simulink model "sampleModel15088_1"  (R2023b)
settings: Solver=VariableStepAuto  StartTime=0.0  StopTime=10.0  RelTol=1e-3
libraries: hdlsllib x4
settings Model: Creator=Tsmc  LastModifiedBy=Tsmc

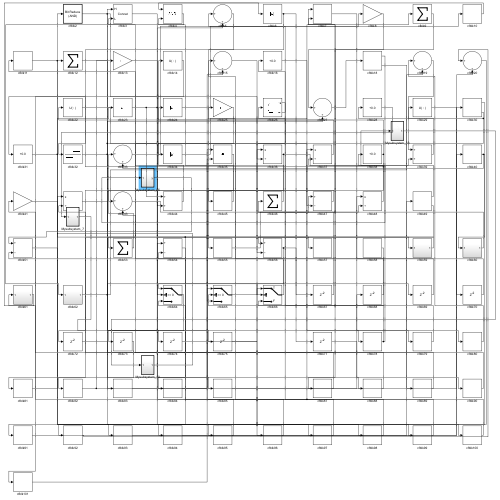
[thumbnail: Simulink's stored preview of the top-level diagram]
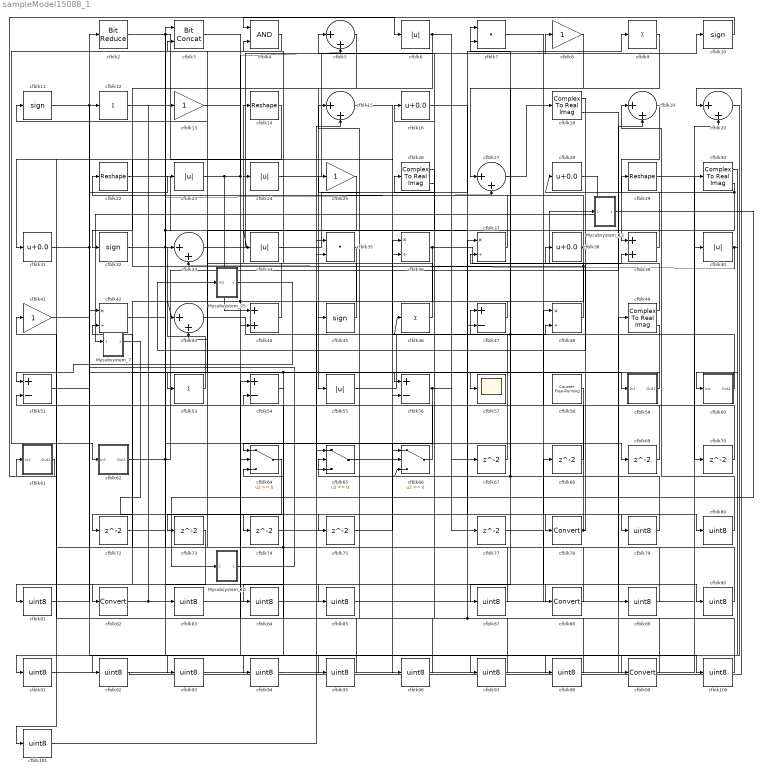
== system sampleModel15088_1 ==
  Mysubsystem_10 : Subsystem  TreatAsAtomicUnit=on  RTWFcnName=Mysubsystem_10
      settings: RTWFcnNameOpts=User specified  RTWFileNameOpts=Use function name
  Mysubsystem_13 : Subsystem  TreatAsAtomicUnit=on  RTWFcnName=Mysubsystem_13
      settings: RTWFcnNameOpts=User specified  RTWFileNameOpts=Use function name
  Mysubsystem_25 : Subsystem  TreatAsAtomicUnit=on  RTWFcnName=Mysubsystem_25
      settings: RTWFcnNameOpts=User specified  RTWFileNameOpts=Use function name
  Mysubsystem_7 : Subsystem  TreatAsAtomicUnit=on  RTWFcnName=Mysubsystem_7
      settings: RTWFcnNameOpts=User specified  RTWFileNameOpts=Use function name
  cfblk{10..11,32,45} (4 alike) : Signum
  cfblk{79..81,83..85,87,89..98,100..101} (19 alike) : DataTypeConversion  OutDataTypeStr=uint8  SaturateOnIntegerOverflow=off  RndMeth=Floor
  cfblk{9,12,46,53} (4 alike) : Sum  Inputs=+
  cfblk{8,13,25,41} (4 alike) : Gain
  cfblk14 : Reshape
  cfblk{5,15,19..20,27,33,43} (7 alike) : Sum  Inputs=|++
  cfblk{16,28,31,38} (4 alike) : Bias  Bias=0.0  SaturateOnIntegerOverflow=off
  cfblk{18,26,30,49} (4 alike) : ComplexToRealImag
  cfblk2 : hdlsllib/Logic and Bit Operations/Bit Reduce  mode=AND
  cfblk22 : Reshape
  cfblk{6,23..24,34,40,55} (6 alike) : Abs  SaturateOnIntegerOverflow=off
  cfblk29 : Reshape
  cfblk3 : hdlsllib/Logic and Bit Operations/Bit Concat  numInputs=2
  cfblk35 : DotProduct  OutDataTypeStr=Inherit: Inherit via internal rule
  cfblk{36..37,42,48} (4 alike) : Product  Inputs=*/  RndMeth=Zero  SaturateOnIntegerOverflow=on
  cfblk39 : Sum
  cfblk4 : Logic  AllPortsSameDT=off  OutDataTypeStr=boolean
  cfblk44 : Sum
  cfblk{47,51,54,56} (4 alike) : Sum  Inputs=+-
  cfblk57 : Scope
  cfblk58 : hdlsllib/Sources/Counter Free-Running  NumBits=16  tsamp=-1
  cfblk59 : Subsystem
  cfblk60 : Subsystem
  cfblk61 : Subsystem
  cfblk62 : Subsystem
  cfblk64 : Switch  SaturateOnIntegerOverflow=off  InputSameDT=off
  cfblk65 : Switch  SaturateOnIntegerOverflow=off  InputSameDT=off
  cfblk66 : Switch  SaturateOnIntegerOverflow=off  InputSameDT=off
  cfblk{67..70,72..75,77} (9 alike) : Delay  SampleTime=1
  cfblk7 : DotProduct  OutDataTypeStr=Inherit: Inherit via internal rule
  cfblk{78,82,88,99} (4 alike) : DataTypeConversion  SaturateOnIntegerOverflow=off  RndMeth=Floor
  wires:
  cfblk33/1 -> cfblk8/1
  cfblk48/1 -> cfblk31/1, cfblk7/2
  cfblk55/1 -> cfblk47/1
  cfblk4/1 -> cfblk62/1(In1)
  cfblk6/1 -> cfblk55/1, cfblk77/1
  cfblk19/1 -> cfblk39/1
  cfblk44/1 -> cfblk14/1
  cfblk53/1 -> cfblk33/1
  cfblk40/1 -> cfblk33/2, cfblk60/1(In1)
  cfblk61/1(Out1) -> cfblk6/1
  cfblk27/1 -> cfblk18/1
  cfblk22/1 -> cfblk47/2
  cfblk37/1 -> cfblk24/1
  cfblk24/1 -> cfblk10/1
  cfblk38/1 -> cfblk22/1, cfblk65/3
  cfblk5/1 -> cfblk32/1
  cfblk31/1 -> cfblk23/1, cfblk57/1
  cfblk59/1(Out1) -> cfblk56/1
  cfblk66/1 -> cfblk25/1
  cfblk60/1(Out1) -> cfblk46/1, cfblk7/1
  cfblk11/1 -> cfblk2/1, cfblk93/1
  cfblk43/1 -> cfblk48/2
  cfblk39/1 -> cfblk29/1
  cfblk46/1 -> cfblk11/1
  cfblk62/1(Out1) -> cfblk19/2, cfblk66/2
  cfblk16/1 -> cfblk78/1
  cfblk36/1 -> cfblk43/1, cfblk44/2, cfblk39/2
  cfblk9/1 -> cfblk27/1
  cfblk25/1 -> cfblk53/1
  cfblk56/1 -> cfblk67/1, cfblk84/1
  cfblk10/1 -> cfblk4/1
  cfblk35/1 -> cfblk82/1
  cfblk32/1 -> cfblk34/1, cfblk27/2, cfblk95/1
  cfblk34/1 -> cfblk9/1
  cfblk3/1 -> cfblk88/1
  cfblk2/1 -> cfblk56/2, cfblk75/1
  cfblk30/2 -> cfblk28/1, cfblk64/2
  cfblk23/1 -> cfblk59/1(In1), cfblk5/2, cfblk44/1
  cfblk26/1 -> cfblk36/2
  cfblk45/1 -> cfblk4/2
  cfblk26/2 -> cfblk5/1
  cfblk47/1 -> cfblk45/1
  cfblk15/1 -> cfblk99/1
  cfblk58/1 -> cfblk65/2
  cfblk49/2 -> cfblk64/1, cfblk72/1
  cfblk67/1 -> cfblk36/1
  cfblk68/1 -> cfblk43/2
  cfblk65/1 -> cfblk69/1
  cfblk69/1 -> cfblk48/1
  cfblk29/1 -> cfblk70/1
  cfblk70/1 -> cfblk51/2
  cfblk64/1 -> cfblk73/1
  cfblk74/1 -> cfblk66/1
  cfblk78/1 -> cfblk37/2, cfblk66/3, cfblk38/1
  cfblk7/1 -> cfblk79/1
  cfblk79/1 -> cfblk16/1
  cfblk12/1 -> cfblk80/1
  cfblk80/1 -> cfblk19/1
  cfblk14/1 -> cfblk81/1
  cfblk81/1 -> cfblk12/1
  cfblk82/1 -> cfblk68/1, cfblk13/1
  cfblk72/1 -> cfblk83/1
  cfblk83/1 -> cfblk35/1
  cfblk84/1 -> cfblk35/2
  cfblk42/1 -> cfblk85/1
  cfblk85/1 -> cfblk30/1
  cfblk8/1 -> cfblk87/1
  cfblk87/1 -> cfblk42/2
  cfblk88/1 -> cfblk64/3, cfblk61/1(In1)
  cfblk18/2 -> cfblk89/1
  cfblk89/1 -> cfblk3/1
  cfblk77/1 -> cfblk90/1
  cfblk90/1 -> cfblk3/2
  cfblk20/1 -> cfblk91/1
  cfblk91/1 -> cfblk49/1
  cfblk30/1 -> cfblk92/1
  cfblk92/1 -> cfblk20/1
  cfblk93/1 -> cfblk20/2
  cfblk54/1 -> cfblk94/1
  cfblk94/1 -> cfblk40/1
  cfblk95/1 -> cfblk54/1
  cfblk75/1 -> cfblk96/1
  cfblk96/1 -> cfblk54/2
  cfblk41/1 -> cfblk97/1
  cfblk97/1 -> cfblk26/1
  cfblk51/1 -> cfblk98/1
  cfblk98/1 -> cfblk41/1
  cfblk99/1 -> cfblk37/1, cfblk65/1
  cfblk13/1 -> cfblk100/1
  cfblk100/1 -> cfblk15/1
  cfblk73/1 -> cfblk101/1
  cfblk101/1 -> cfblk15/2
  cfblk28/1 -> Mysubsystem_7/1(In1)
  Mysubsystem_7/1(Out1) -> cfblk74/1
  Mysubsystem_10/1(Out1) -> cfblk42/1
  cfblk49/1 -> Mysubsystem_13/1(In1)
  Mysubsystem_13/1(Out1) -> Mysubsystem_10/1(In1)
  cfblk18/1 -> Mysubsystem_25/1(In1)
  Mysubsystem_25/1(y) -> cfblk51/1

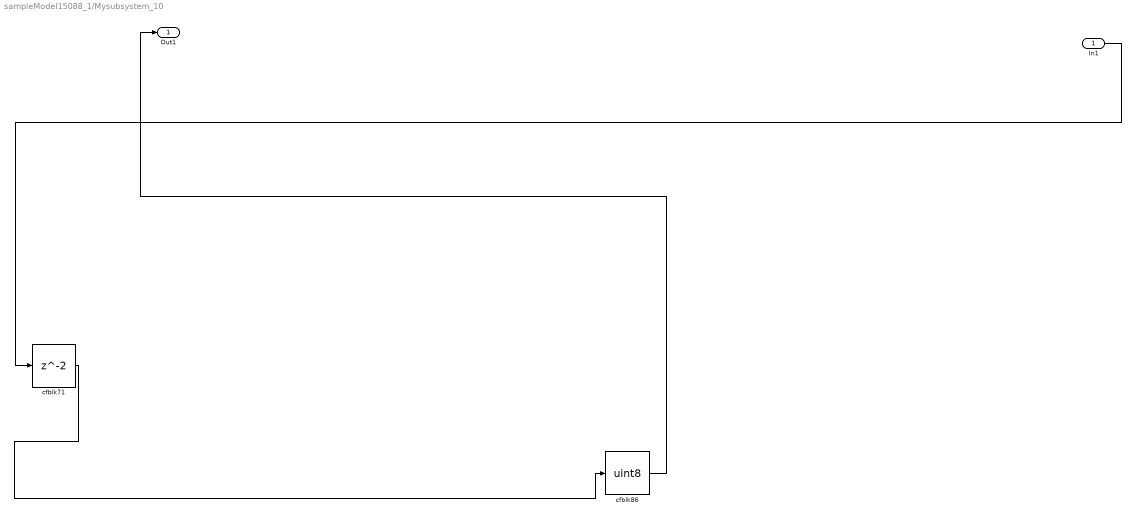
== system sampleModel15088_1/Mysubsystem_10 ==
  In1 : Inport
  cfblk71 : Delay  SampleTime=1
  cfblk86 : DataTypeConversion  OutDataTypeStr=uint8  SaturateOnIntegerOverflow=off  RndMeth=Floor
  Out1 : Outport
  wires:
  cfblk71/1 -> cfblk86/1
  In1/1 -> cfblk71/1
  cfblk86/1 -> Out1/1

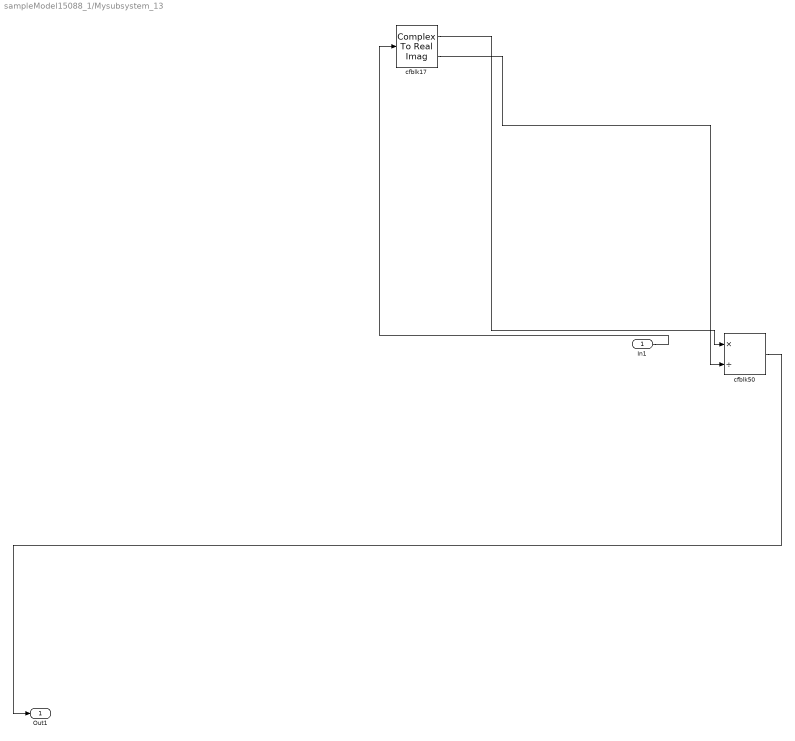
== system sampleModel15088_1/Mysubsystem_13 ==
  In1 : Inport
  cfblk17 : ComplexToRealImag
  cfblk50 : Product  Inputs=*/  RndMeth=Zero  SaturateOnIntegerOverflow=on
  Out1 : Outport
  wires:
  cfblk17/1 -> cfblk50/1
  cfblk17/2 -> cfblk50/2
  cfblk50/1 -> Out1/1
  In1/1 -> cfblk17/1

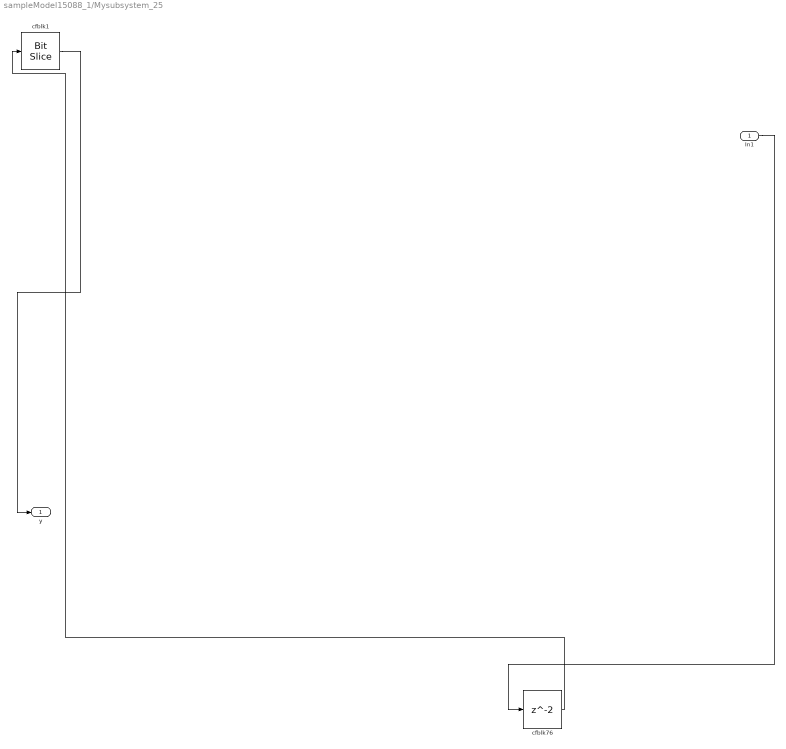
== system sampleModel15088_1/Mysubsystem_25 ==
  In1 : Inport
  cfblk1 : hdlsllib/Logic and Bit Operations/Bit Slice  lidx=7  ridx=0
  cfblk76 : Delay  SampleTime=1
  y : Outport
  wires:
  cfblk76/1 -> cfblk1/1
  In1/1 -> cfblk76/1
  cfblk1/1 -> y/1

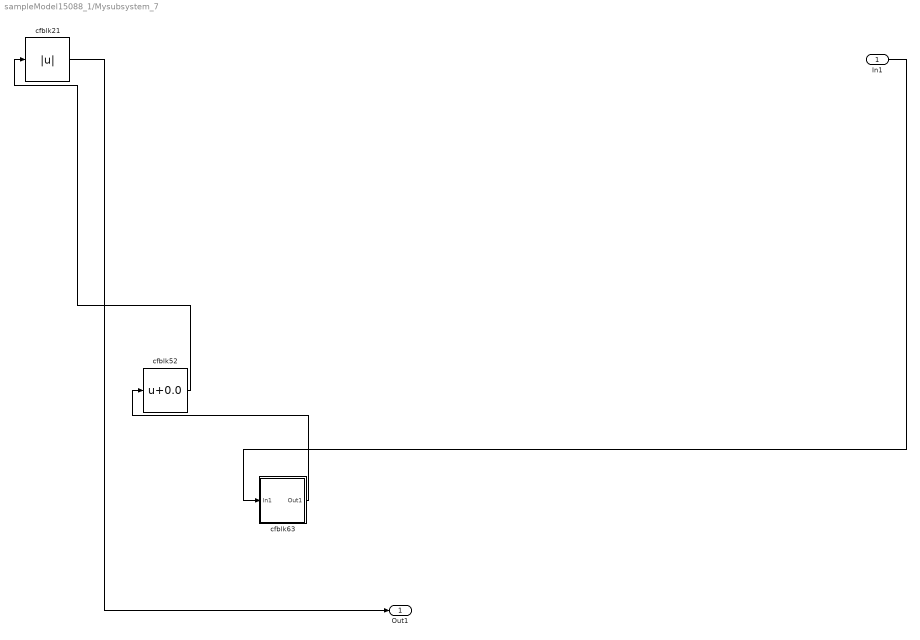
== system sampleModel15088_1/Mysubsystem_7 ==
  In1 : Inport
  cfblk21 : Abs  SaturateOnIntegerOverflow=off
  cfblk52 : Bias  Bias=0.0  SaturateOnIntegerOverflow=off
  cfblk63 : Subsystem
  Out1 : Outport
  wires:
  cfblk52/1 -> cfblk21/1
  cfblk63/1(Out1) -> cfblk52/1
  cfblk21/1 -> Out1/1
  In1/1 -> cfblk63/1(In1)

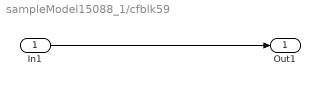
== system sampleModel15088_1/cfblk59 ==
  In1 : Inport
  Out1 : Outport
  wires:
  In1/1 -> Out1/1

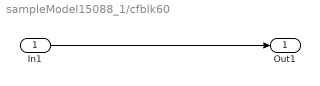
== system sampleModel15088_1/cfblk60 ==
  In1 : Inport
  Out1 : Outport
  wires:
  In1/1 -> Out1/1

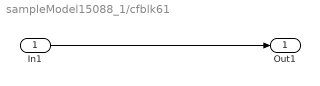
== system sampleModel15088_1/cfblk61 ==
  In1 : Inport
  Out1 : Outport
  wires:
  In1/1 -> Out1/1

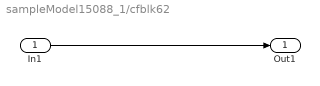
== system sampleModel15088_1/cfblk62 ==
  In1 : Inport
  Out1 : Outport
  wires:
  In1/1 -> Out1/1

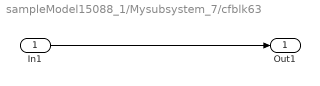
== system sampleModel15088_1/Mysubsystem_7/cfblk63 ==
  In1 : Inport
  Out1 : Outport
  wires:
  In1/1 -> Out1/1
